simulink model "PID_controlinput_disturbance"  (R2022a)
settings: Solver=VariableStepAuto  StartTime=0.0  StopTime=0.05  RelTol=1e-3
libraries: cstblocks x2
settings Model: Creator=Linxi Ren  LastModifiedBy=Linxi Ren

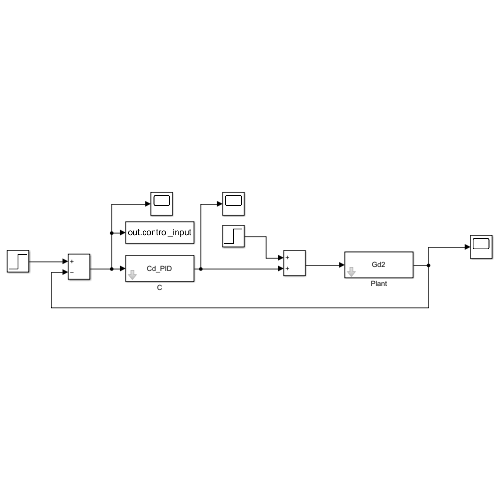
[thumbnail: Simulink's stored preview of the top-level diagram]
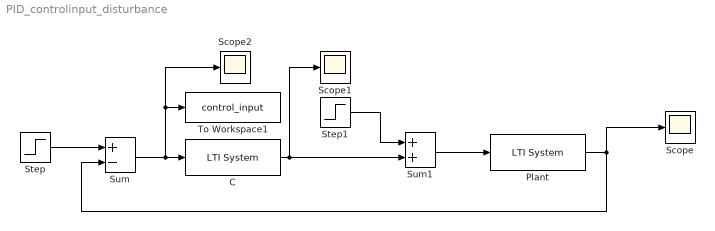
== system PID_controlinput_disturbance ==
  C : cstblocks/LTI System  sys=Cd_PID  IC=[]
  Plant : cstblocks/LTI System  sys=Gd2  IC=[]
  Scope : Scope
  Scope1 : Scope
  Scope2 : Scope
  Step : Step  Time=0  After=0  SampleTime=0
  Step1 : Step  Time=0  SampleTime=0.0005
  Sum : Sum  Inputs=+-  InputSameDT=on  SaturateOnIntegerOverflow=on  OutDataTypeStr=Inherit: Same as first input
  Sum1 : Sum  InputSameDT=on  SaturateOnIntegerOverflow=on  OutDataTypeStr=Inherit: Same as first input
  To Workspace1 : ToWorkspace  VariableName=control_input  SaveFormat=Timeseries  SampleTime=-1
  wires:
  Sum/1 -> Scope2/1, To Workspace1/1, C/1
  Step1/1 -> Sum1/1
  Plant/1 -> Sum/2, Scope/1
  Sum1/1 -> Plant/1
  C/1 -> Sum1/2, Scope1/1
  Step/1 -> Sum/1
